simulink model "Sistemul_incalzire_pardoseala"  (R2021b)
settings: Solver=VariableStepAuto  StartTime=0.0  StopTime=10000  RelTol=1e-3
values from neighbouring files (symbols this model uses):
  A = [-1/Ta -ke/La;km/J 0]    [valori_mcc.m]    (also in valori_sistem_de_incazire_pardoseala.m = [-1/Tp 1/Tp;kp/(kc*Tc) -((1+kp/kc)/Tc)])
  B = [kE/La 0;0 -1/J]    [valori_mcc.m]    (also in valori_sistem_de_incazire_pardoseala.m = [kE/(kp*Tp) 0;0 1/Tc])
  C = [1 0;0 1]    [valori_mcc.m]    (also in valori_sistem_de_incazire_pardoseala.m = [0 1])
  D = [0 0;0 0]    [valori_mcc.m]    (also in valori_sistem_de_incazire_pardoseala.m = [0 0])
  kc = 125    [valori_sistem_de_incazire_pardoseala.m]
  kE = 42.85    [valori_mcc.m]    (also in valori_sistem_de_incazire_pardoseala.m = 1000)
  kp = 500    [valori_sistem_de_incazire_pardoseala.m]
  Tc = 300    [valori_sistem_de_incazire_pardoseala.m]
  Tp = 60    [valori_sistem_de_incazire_pardoseala.m]
settings Model: Creator=alexandra.szedlak-st  LastModifiedBy=alexandra.szedlak-st

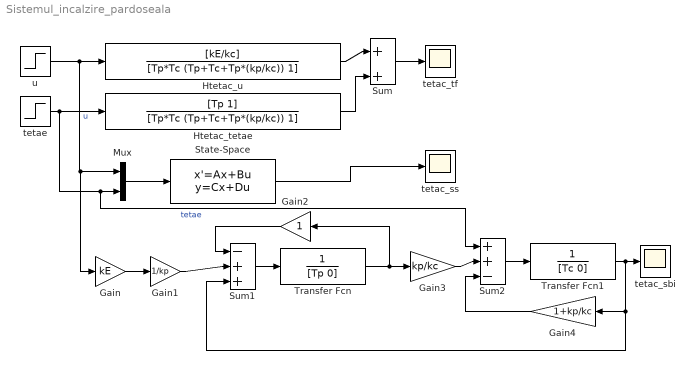
== system Sistemul_incalzire_pardoseala ==
  Gain : Gain  Gain=kE
  Gain1 : Gain  Gain=1/kp
  Gain2 : Gain
  Gain3 : Gain  Gain=kp/kc
  Gain4 : Gain  Gain=1+kp/kc
  Htetac_tetae : TransferFcn  Numerator=[Tp 1]  Denominator=[Tp*Tc (Tp+Tc+Tp*(kp/kc)) 1]
  Htetac_u : TransferFcn  Numerator=[kE/kc]  Denominator=[Tp*Tc (Tp+Tc+Tp*(kp/kc)) 1]
  Mux : Mux  Inputs=2
  State-Space : StateSpace  A=A  B=B  C=C  D=D  InitialCondition=0
  Sum : Sum  Inputs=|++
  Sum1 : Sum  Inputs=|-++
  Sum2 : Sum  Inputs=|++-
  Transfer Fcn : TransferFcn  Denominator=[Tp 0]
  Transfer Fcn1 : TransferFcn  Denominator=[Tc 0]
  tetac_sbi : Scope
  tetac_ss : Scope
  tetac_tf : Scope
  tetae : Step  Time=5000  After=-10  SampleTime=0
  u : Step  Time=0  After=2.5  SampleTime=0
  wires:
  u/1 -> Gain/1, Mux/1, Htetac_u/1  "u"
  tetae/1 -> Sum2/1, Mux/2, Htetac_tetae/1  "tetae"
  Htetac_u/1 -> Sum/1
  Htetac_tetae/1 -> Sum/2
  Sum/1 -> tetac_tf/1
  State-Space/1 -> tetac_ss/1
  Mux/1 -> State-Space/1
  Gain/1 -> Gain1/1
  Gain1/1 -> Sum1/2
  Gain2/1 -> Sum1/1
  Sum1/1 -> Transfer Fcn/1
  Transfer Fcn/1 -> Gain3/1, Gain2/1
  Gain3/1 -> Sum2/2
  Sum2/1 -> Transfer Fcn1/1
  Transfer Fcn1/1 -> Sum1/3, Gain4/1, tetac_sbi/1
  Gain4/1 -> Sum2/3
